simulink model "obstacleStopper"  (R2019b)
settings: Solver=FixedStepAuto  StartTime=0.0  StopTime=inf  FixedStep=0.02  RelTol=1e-3  EnableMultiTasking=on
undefined symbols (not defined in the file): Angular, Linear
libraries: robotlib x5
settings Model: Creator=sprinkle  LastModifiedBy=ivory
settings DataIOCC: ReturnWorkspaceOutputs=off
settings OptimizationCC: LifeSpan=Inf  MaxStackSize=64  EfficientTunableParamExpr=on
settings DebuggingCC: SFUnexpectedBacktrackingDiag=warning  SFNoUnconditionalDefaultTransitionDiag=warning  SFExecutionAtInitializationDiag=none  ArithmeticOperatorsInVariantConditions=warning
settings HardwareCC: ProdBitPerPointer=32  ProdBitPerSizeT=32  ProdBitPerPtrDiffT=32  ProdLargestAtomicFloat=None  ProdIntDivRoundTo=Undefined  ProdEndianess=Unspecified  ProdWordSize=32  ProdHWDeviceType=Generic->Unspecified (assume 32-bit Generic)
settings SFSimCC: SimUseLocalCustomCode=off  MATLABDynamicMemAlloc=off  CustomCodeUndefinedFunction=UseInterfaceOnly
settings RTWCC: SystemTargetFile=ert.tlc  HardwareBoard=Robot Operating System (ROS)  TLCOptions=-aInlineSetEventsForThisBaseRateFcn=TLC_FALSE -aSuppressMultiTaskScheduler=TLC_FALSE -aRateBasedStepFcn=0  TemplateMakefile=ert_default_tmf  GenerateReport=on  RTWUseLocalCustomCode=off  Toolchain=Catkin  IncludeHyperlinkInReport=on  LaunchReport=on  TargetLang=C++  GenerateTraceInfo=on  GenerateTraceReport=on  GenerateTraceReportSl=on  GenerateTraceReportSf=on  GenerateTraceReportEml=on
settings CodeAppCC: ForceParamTrailComments=on  IgnoreCustomStorageClasses=off  OperatorAnnotations=on  SimulinkDataObjDesc=on  SFDataObjDesc=on  MATLABFcnDesc=on  InsertBlockDesc=on  StateflowObjectComments=on  MATLABSourceComments=on
settings ERTTargetCC: MultiwordLength=2048
settings ConfigComp: CovMetricSettings=dw  CovHtmlReporting=on  CovSaveCumulativeToWorkspaceVar=on  CovSaveSingleToWorkspaceVar=on  CovExternalEMLEnable=off

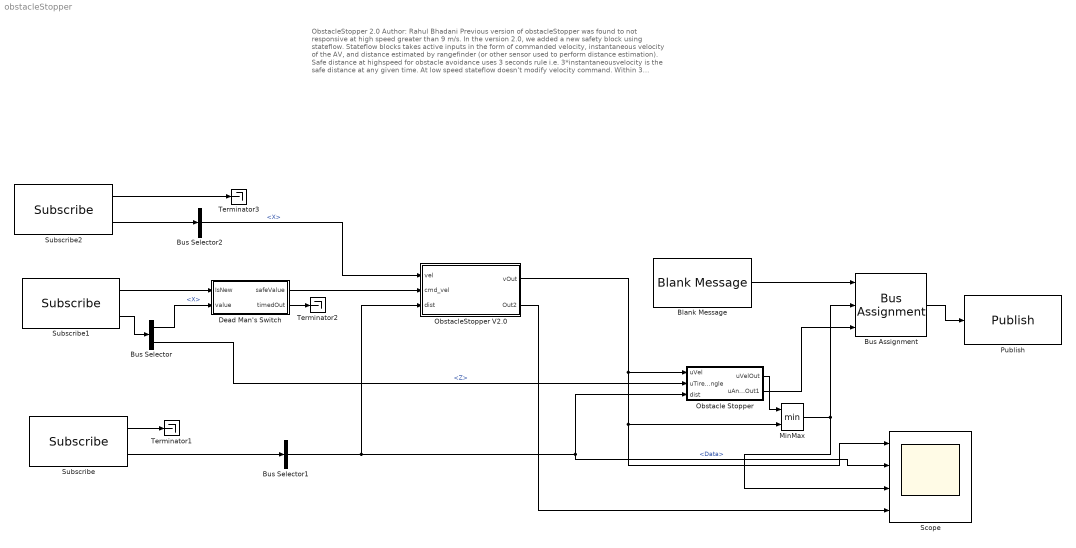
== system obstacleStopper ==
  note: ObstacleStopper 2.0
      | Author: Rahul Bhadani
      | Previous version of obstacleStopper was found to not responsive at
      | high speed greater than 9 m/s. In the version 2.0, we added a new safety block
      | using stateflow. Stateflow blocks takes active inputs in the form of commanded
      | velocity, instantaneous velocity of the AV, and distance estimated by
      | rangefinder (or other sensor used to perform distance estimation).
      | Safe distance at highspeed for obstacle avoidance uses 3 seconds rule i.e.
      | 3*instantaneousvelocity is the safe distance at any given time. At low speed
      | stateflow doesn't modify velocity command. Within 3 seconds distance, the stateflow
      | start reducing velocity of the AV by factor of 10 to mimick hardbraking.
  Blank Message : robotlib/Blank Message  messageClass=Message  entityType=geometry_msgs/Twist  messageType=geometry_msgs/Twist  SampleTime=inf
      settings: SourceProductBaseCode=RO
  Bus Assignment : BusAssignment  AssignedSignals=Linear.X,Angular.Z
  Bus Selector : BusSelector  OutputSignals=Linear.X,Angular.Z
  Bus Selector1 : BusSelector  OutputSignals=Data
  Bus Selector2 : BusSelector  OutputSignals=Linear.X
  Dead Man's Switch : Subsystem  TreatAsAtomicUnit=on  mask{stepSize=0.02, timeout=0.2}
      mask prompts: stepSize "Simulation step size"; timeout "Timeout (in seconds)"
      mask help: Interprets whether a new message has been recently received, and if so permits the data in 'value' to be passed through. Otherwise, 0 is outputted from 'safeValue'
      mask Help: Interprets whether a new message has been recently received, and if so permits the data in 'value' to be passed through. Otherwise, 0 is outputted from 'safeValue'
  MinMax : MinMax  Inputs=2
  Obstacle Stopper : Subsystem
  ObstacleStopper V2.0 : Subsystem
  Publish : robotlib/Publish  topicSource=Specify your own  topic=cmd_vel_safe  messageType=geometry_msgs/Twist  messageQueueLength=1
      settings: SourceProductBaseCode=RO
  Scope : Scope  NumInputPorts=4
  Subscribe : robotlib/Subscribe  topicSource=Specify your own  topic=distanceEstimatorSteeringBased/dist  messageType=std_msgs/Float64  sampleTime=-1  messageQueueLength=1
      settings: SourceProductBaseCode=RO
  Subscribe1 : robotlib/Subscribe  topicSource=Specify your own  topic=cmd_vel  messageType=geometry_msgs/Twist  sampleTime=-1  messageQueueLength=1
      settings: SourceProductBaseCode=RO
  Subscribe2 : robotlib/Subscribe  topicSource=Specify your own  topic=vel  messageType=geometry_msgs/Twist  sampleTime=-1  messageQueueLength=1
      settings: SourceProductBaseCode=RO
  Terminator1 : Terminator
  Terminator2 : Terminator
  Terminator3 : Terminator
  wires:
  Subscribe1/2 -> Bus Selector/1
  Subscribe1/1 -> Dead Man's Switch/1(IsNew)
  Bus Selector/2 -> Obstacle Stopper/2(uTireAngle)  "<Z>"
  Blank Message/1 -> Bus Assignment/1
  Bus Assignment/1 -> Publish/1
  Obstacle Stopper/2(uAngleOut1) -> Bus Assignment/3
  Subscribe/1 -> Terminator1/1
  Subscribe/2 -> Bus Selector1/1
  Bus Selector1/1 -> Scope/2, Obstacle Stopper/3(dist), ObstacleStopper V2.0/3(dist)  "<Data>"
  Bus Selector/1 -> Dead Man's Switch/2(value)  "<X>"
  Dead Man's Switch/2(timedOut) -> Terminator2/1
  MinMax/1 -> Bus Assignment/2, Scope/3
  Obstacle Stopper/1(uVelOut) -> MinMax/1
  Subscribe2/1 -> Terminator3/1
  Subscribe2/2 -> Bus Selector2/1
  ObstacleStopper V2.0/1(vOut) -> MinMax/2, Scope/1, Obstacle Stopper/1(uVel)
  Bus Selector2/1 -> ObstacleStopper V2.0/1(vel)  "<X>"
  Dead Man's Switch/1(safeValue) -> ObstacleStopper V2.0/2(cmd_vel)
  ObstacleStopper V2.0/2(Out2) -> Scope/4

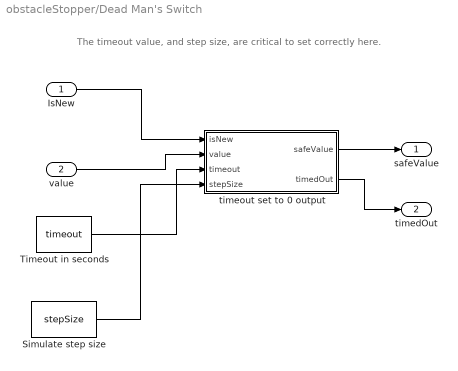
== system obstacleStopper/Dead Man's Switch ==
  note: The timeout value, and step size, are critical to set correctly here.
  IsNew : Inport
  value : Inport  Port=2
  Simulate step size : Constant  Value=stepSize
  Timeout in seconds : Constant  Value=timeout
  timeout set to 0 output : MATLAB Function  TreatAsAtomicUnit=on
  safeValue : Outport  InitialOutput=[0]  VectorParamsAs1DForOutWhenUnconnected=off
  timedOut : Outport  Port=2  InitialOutput=[0]  VectorParamsAs1DForOutWhenUnconnected=off
  wires:
  IsNew/1 -> timeout set to 0 output/1(isNew)
  timeout set to 0 output/1(safeValue) -> safeValue/1
  value/1 -> timeout set to 0 output/2(value)
  Timeout in seconds/1 -> timeout set to 0 output/3(timeout)
  timeout set to 0 output/2(timedOut) -> timedOut/1
  Simulate step size/1 -> timeout set to 0 output/4(stepSize)

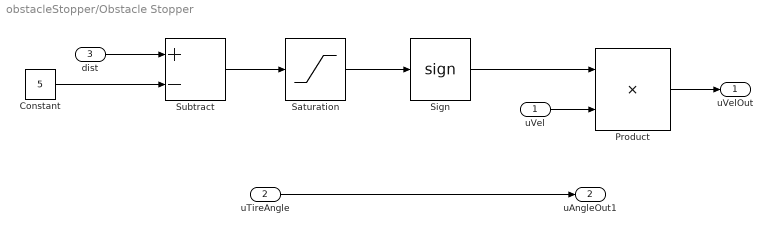
== system obstacleStopper/Obstacle Stopper ==
  uVel : Inport
  uTireAngle : Inport  Port=2
  dist : Inport  Port=3
  Constant : Constant  Value=5
  Product : Product
  Saturation : Saturate  UpperLimit=1  LowerLimit=0
  Sign : Signum
  Subtract : Sum  Inputs=+-
  uVelOut : Outport  VectorParamsAs1DForOutWhenUnconnected=off
  uAngleOut1 : Outport  Port=2  VectorParamsAs1DForOutWhenUnconnected=off
  wires:
  Constant/1 -> Subtract/2
  dist/1 -> Subtract/1
  Subtract/1 -> Saturation/1
  Saturation/1 -> Sign/1
  uVel/1 -> Product/2
  Sign/1 -> Product/1
  Product/1 -> uVelOut/1
  uTireAngle/1 -> uAngleOut1/1

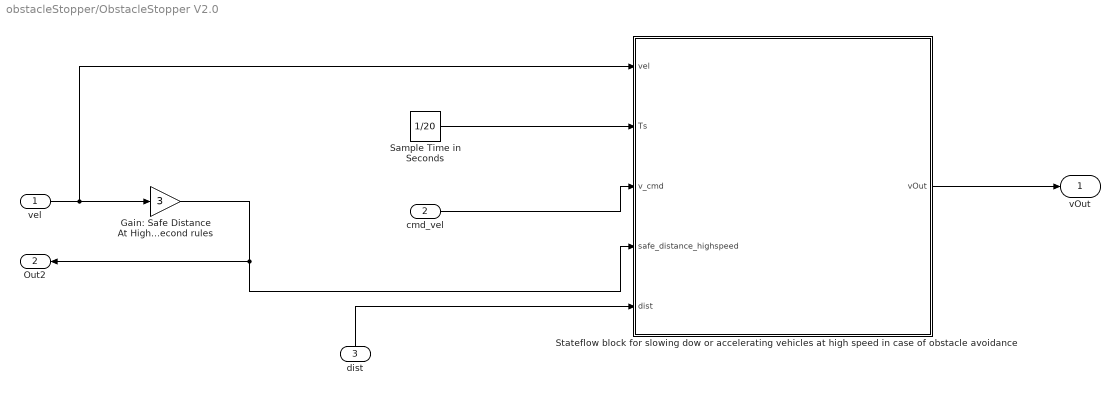
== system obstacleStopper/ObstacleStopper V2.0 ==
  vel : Inport
  cmd_vel : Inport  Port=2
  dist : Inport  Port=3
  Gain: Safe Distance At HighSpeed follows 3 second rules : Gain  Gain=3
  Sample Time in Seconds : Constant  Value=1/20
  Stateflow block for slowing dow or accelerating vehicles at high speed in case of obstacle avoidance : Stateflow chart  TreatAsAtomicUnit=on
  vOut : Outport  VectorParamsAs1DForOutWhenUnconnected=off
  Out2 : Outport  Port=2  VectorParamsAs1DForOutWhenUnconnected=off
  wires:
  dist/1 -> Stateflow block for slowing dow or accelerating vehicles at high speed in case of obstacle avoidance/5(dist)
  Stateflow block for slowing dow or accelerating vehicles at high speed in case of obstacle avoidance/1(vOut) -> vOut/1
  cmd_vel/1 -> Stateflow block for slowing dow or accelerating vehicles at high speed in case of obstacle avoidance/3(v_cmd)
  vel/1 -> Gain: Safe Distance At HighSpeed follows 3 second rules/1, Stateflow block for slowing dow or accelerating vehicles at high speed in case of obstacle avoidance/1(vel)
  Sample Time in Seconds/1 -> Stateflow block for slowing dow or accelerating vehicles at high speed in case of obstacle avoidance/2(Ts)
  Gain: Safe Distance At HighSpeed follows 3 second rules/1 -> Out2/1, Stateflow block for slowing dow or accelerating vehicles at high speed in case of obstacle avoidance/4(safe_distance_highspeed)

== stateflow chart obstacleStopper/ObstacleStopper V2.0/Stateflow block for slowing dow or accelerating vehicles at high speed in case of obstacle avoidance ==
  state Check_initial_Safe_distance
    entry:distance = dist;
    during:vOut = 0;
  note: If initial distance is less than 3 second distance,
      | then command velocity  equal to one third of
      | originally commanded velocity.
  state NormalDrive
    entry: vOut = v_cmd; distance = dist;
    during: vOut = v_cmd; distance = dist;
  state NewCommand
    entry:  vOut = v_cmd/3; distance = dist;
    during: vOut = v_cmd/3; distance = dist;
  state Decelerate
    entry:  vOut = vel/10; distance = dist;
    during: vOut = vel/10; distance = dist;
  state Accelerate
    entry: count = 1
    during: vOut = vel + 0.05*(Ts); count = count + 1;
  (default) -> Check_initial_Safe_distance
  Check_initial_Safe_distance -> NewCommand [order 2] : [distance  <= 3*v_cmd]
  Check_initial_Safe_distance -> NormalDrive [order 1] : [distance > (3*v_cmd)]
  Decelerate -> Decelerate [order 2] : [distance < safe_distance_highspeed]
  NewCommand -> NormalDrive : [distance >= safe_distance_highspeed]
  NormalDrive -> Decelerate [order 1] : [distance < safe_distance_highspeed && vel >= 9]
  Accelerate -> NormalDrive [order 2] : [count >=(1/Ts) || vOut >= v_cmd]
  NormalDrive -> NormalDrive [order 2] : [distance >= safe_distance_highspeed ||  vel < 9]
  Decelerate -> Accelerate [order 1] : [distance >= safe_distance_highspeed]
  Accelerate -> Accelerate [order 1] : [count <(1/Ts) && vOut < v_cmd]
  data: vOut output; vel input; Ts input; v_cmd input; safe_distance_highspeed input; count local; dist input; distance local

== matlab function obstacleStopper/Dead Man's Switch/timeout set to 0 output ==
  data: isNew input; safeValue output; value input; timeout input; timedOut output; stepSize input
function [safeValue,timedOut] = fcn(isNew,value,timeout,stepSize)
%#codegen
persistent sinceLastMsg
timedOut=true;
if isempty(sinceLastMsg)
    sinceLastMsg=(timeout/stepSize)+1;
end

safeValue=0;
% if no new message
% after timeout, we output 0
if( isNew == true )
    sinceLastMsg = 0;
else
    sinceLastMsg = sinceLastMsg+1;
end

% Note: we require step size as an input here, and depend on our
% system being executed at a regular rate, or bad things will happen
if( sinceLastMsg < timeout/stepSize )
    timedOut = false;
end
    
if( timedOut == false )
    safeValue = value;
end
